simulink model "model"  (R2022a)
settings: Solver=VariableStepAuto  StartTime=0.0  StopTime=0.002  RelTol=1e-3
values from neighbouring files (symbols this model uses):
  c1 = 220e-6    (= 0.00022)    [Untitled.m]
  c2 = 220e-6    (= 0.00022)    [Untitled.m]
  lb = 33e-6    (= 3.3e-05)    [Untitled.m]
  lr = 1.7e-6    (= 1.7e-06)    [Untitled.m]
  rb = 0.010    (= 0.01)    [Untitled.m]
  sc1 = 0.350    (= 0.35)    [Untitled.m]
  sc2 = 0.350    (= 0.35)    [Untitled.m]
  vb = 3.3    [Untitled.m]
  w = 2*pi*20e3    (= 125663.706144)    [Untitled.m]
libraries: spsSeriesRLCBranchLib x8, spsIdealSwitchLib x4, spsVoltageMeasurementLib x2, spsCurrentMeasurementLib x1, spsDCVoltageSourceLib x1, spspowerguiLib x1
settings Model: Creator=nunin  LastModifiedBy=up201806419
settings SolverCC: AlgebraicLoopSolver=TrustRegion
settings DebuggingCC: UnconnectedInputMsg=warning  UnconnectedOutputMsg=warning  UnconnectedLineMsg=warning  SFMachineParentedDataDiag=warning

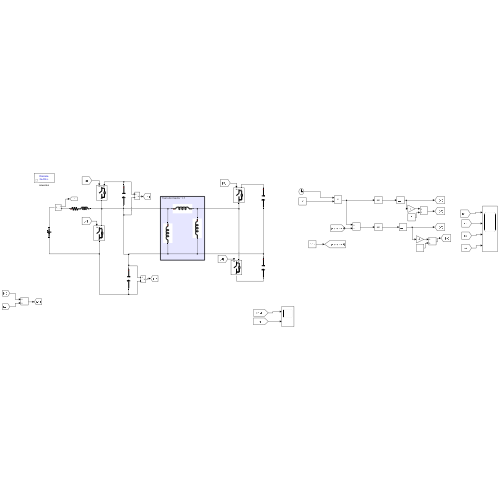
[thumbnail: Simulink's stored preview of the top-level diagram]
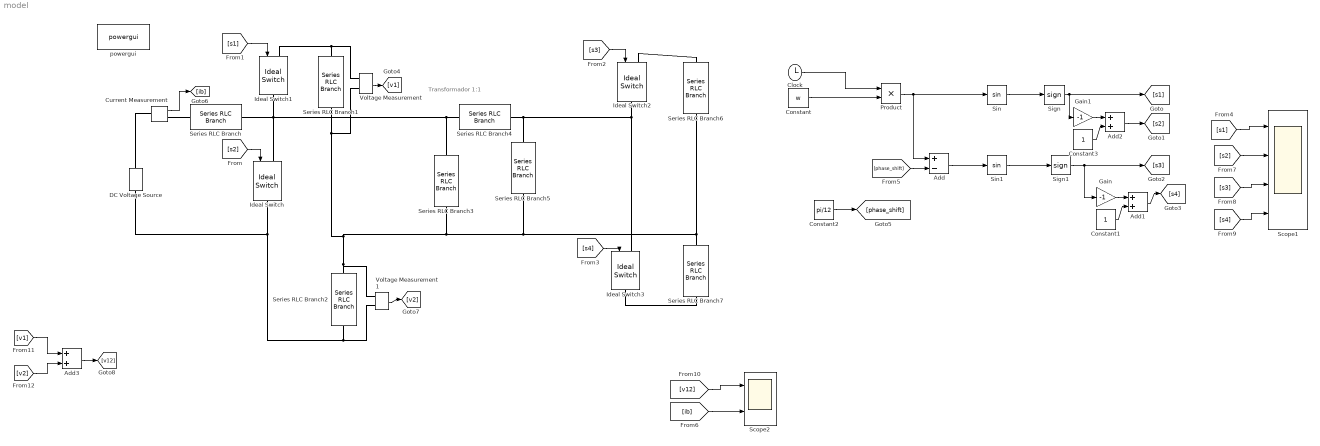
== system model ==
  note: Transformador 1:1
  Add : Sum  Inputs=+-
  Add1 : Sum
  Add2 : Sum
  Add3 : Sum
  Clock : Clock
  Constant : Constant  Value=w
  Constant1 : Constant
  Constant2 : Constant  Value=pi/12
  Constant3 : Constant
  Current Measurement : spsCurrentMeasurementLib/Current Measurement  PhasorSimulation=off  OutputType=Complex  PSBequivalent=0
  DC Voltage Source : spsDCVoltageSourceLib/DC Voltage Source  Amplitude=vb  Measurements=None
  Gain : Gain  Gain=-1
  Gain1 : Gain  Gain=-1
  Ideal Switch{,1..3} (4 alike) : spsIdealSwitchLib/Ideal Switch  Ron=0.001  Lon=0  IC=0  Rs=1e5  Cs=inf  Measurements=off
  Product : Product
  Scope1 : Scope  NumInputPorts=4
  Scope2 : Scope  NumInputPorts=2
  Series RLC Branch : spsSeriesRLCBranchLib/Series RLC Branch  LConnTagsString=__new0  RConnTagsString=__new0  BranchType=RL  Resistance=rb  Inductance=lb  SetiL0=off  InitialCurrent=0  Capacitance=1e-6  Setx0=off  InitialVoltage=0  Measurements=None
  Series RLC Branch1 : spsSeriesRLCBranchLib/Series RLC Branch  LConnTagsString=__new0  RConnTagsString=__new0  BranchType=C  Resistance=rb  Inductance=lb  SetiL0=off  InitialCurrent=0  Capacitance=c1  Setx0=on  InitialVoltage=3.3  Measurements=None
  Series RLC Branch2 : spsSeriesRLCBranchLib/Series RLC Branch  LConnTagsString=__new0  RConnTagsString=__new0  BranchType=C  Resistance=rb  Inductance=lb  SetiL0=off  InitialCurrent=0  Capacitance=c2  Setx0=on  InitialVoltage=3.3  Measurements=None
  Series RLC Branch3 : spsSeriesRLCBranchLib/Series RLC Branch  LConnTagsString=__new0  RConnTagsString=__new0  BranchType=L  Resistance=rb  Inductance=lr/100  SetiL0=off  InitialCurrent=0  Capacitance=1e-6  Setx0=off  InitialVoltage=0  Measurements=None
  Series RLC Branch4 : spsSeriesRLCBranchLib/Series RLC Branch  LConnTagsString=__new0  RConnTagsString=__new0  BranchType=L  Resistance=rb  Inductance=lr  SetiL0=off  InitialCurrent=0  Capacitance=1e-6  Setx0=off  InitialVoltage=0  Measurements=None
  Series RLC Branch5 : spsSeriesRLCBranchLib/Series RLC Branch  LConnTagsString=__new0  RConnTagsString=__new0  BranchType=L  Resistance=rb  Inductance=lr/100  SetiL0=off  InitialCurrent=0  Capacitance=1e-6  Setx0=off  InitialVoltage=0  Measurements=None
  Series RLC Branch6 : spsSeriesRLCBranchLib/Series RLC Branch  LConnTagsString=__new0  RConnTagsString=__new0  BranchType=C  Resistance=rb  Inductance=lb  SetiL0=off  InitialCurrent=0  Capacitance=sc1  Setx0=on  InitialVoltage=3.3  Measurements=None
  Series RLC Branch7 : spsSeriesRLCBranchLib/Series RLC Branch  LConnTagsString=__new0  RConnTagsString=__new0  BranchType=C  Resistance=rb  Inductance=lb  SetiL0=off  InitialCurrent=0  Capacitance=sc2  Setx0=on  InitialVoltage=3.3  Measurements=None
  Sign : Signum  ZeroCross=off
  Sign1 : Signum
  Sin : Trigonometry
  Sin1 : Trigonometry
  Voltage Measurement : spsVoltageMeasurementLib/Voltage Measurement  PhasorSimulation=off  OutputType=Complex  PSBequivalent=0
  Voltage Measurement1 : spsVoltageMeasurementLib/Voltage Measurement  PhasorSimulation=off  OutputType=Complex  PSBequivalent=0
  powergui : spspowerguiLib/powergui  Priority=1  SimulationMode=Discrete  SampleTime=2e-9  frequency=60  Iterations=50  frequencyindice=0  Pbase=100e6  ErrMax=1e-4  UnitsV=kV  UnitsW=MW  buscounter=0  FunctionMessages=off  echomessages=off  EnableUseOfTLC=off  CurrentSourceSwitches=off  DisableSnubberDevices=off  DisableRonSwitches=off  DisableVfSwitches=off  DisplayEquations=off  AutomaticDiscreteSolvers=off  SolverType=Tustin/Backward Euler (TBE)  Interpol=off  ExternalGateDelay=off  methode=off  Ts=100  x0status=blocks  SPID=on  SwTol=0  HookPort=off  NonlinearTolerance=1e-4  nMaxIteration=100  ContinueOnMaxIteration=off  RestoreLinks=warning  ResistiveCurrentMeasurement=off  Frange=[0:2:500]  Ylog=off  Xlog=on  ShowGrid=off  save=off  variable=ZData  structure=0  ZoomFFT=off  StartTime=0.0  cycles=1  DisplayStyle=1  fundamental=60  FreqAxis=off  MaxFrequency=1000  frequencyindicesteady=1  RmsSteady=1  display=off
  wires:
  [s2] -> Ideal Switch/1
  [s1] -> Ideal Switch1/1
  [s3] -> Ideal Switch2/1
  Clock/1 -> Product/1
  Constant/1 -> Product/2
  Product/1 -> Add/1, Sin/1
  [phase_shift] -> Add/2
  Add/1 -> Sin1/1
  Sin/1 -> Sign/1
  Sin1/1 -> Sign1/1
  Sign/1 -> Gain1/1, [s1]
  Add2/1 -> [s2]
  Sign1/1 -> Gain/1, [s3]
  Constant2/1 -> [phase_shift]
  Current Measurement/1 -> [ib]
  [ib] -> Scope2/2
  [s1] -> Scope1/1
  [s2] -> Scope1/2
  [s3] -> Scope1/3
  [s4] -> Scope1/4
  Add1/1 -> [s4]
  Gain/1 -> Add1/1
  Constant1/1 -> Add1/2
  Constant3/1 -> Add2/2
  Gain1/1 -> Add2/1
  Voltage Measurement/1 -> [v1]
  [v12] -> Scope2/1
  Voltage Measurement1/1 -> [v2]
  [v1] -> Add3/1
  [v2] -> Add3/2
  Add3/1 -> [v12]
  [s4] -> Ideal Switch3/1
  connections:
  Series RLC Branch/RConn1 -- Ideal Switch1/RConn1 -- Ideal Switch/LConn1 -- Series RLC Branch4/LConn1 -- Series RLC Branch3/LConn1
  Series RLC Branch1/LConn1 -- Ideal Switch1/LConn1 -- Voltage Measurement/LConn1
  Series RLC Branch5/LConn1 -- Ideal Switch3/LConn1 -- Ideal Switch2/RConn1 -- Series RLC Branch4/RConn1
  Ideal Switch2/LConn1 -- Series RLC Branch6/LConn1
  Ideal Switch3/RConn1 -- Series RLC Branch7/RConn1
  Current Measurement/RConn1 -- Series RLC Branch/LConn1
  Current Measurement/LConn1 -- DC Voltage Source/RConn1
  Voltage Measurement1/LConn2 -- Ideal Switch/RConn1 -- DC Voltage Source/LConn1 -- Series RLC Branch2/RConn1
  Series RLC Branch6/RConn1 -- Series RLC Branch7/LConn1 -- Voltage Measurement1/LConn1 -- Series RLC Branch2/LConn1 -- Voltage Measurement/LConn2 -- Series RLC Branch1/RConn1 -- Series RLC Branch3/RConn1 -- Series RLC Branch5/RConn1
